simulink model "Distribution_v2"  (Simulink 7.9)
settings: Solver=VariableStepDiscrete  StartTime=0.0  StopTime=1000  RelTol=1e-3
libraries: simeventslib x35
(part 4 of 6)

== system Distribution_v2/Transportation_Channel_42 ==
  note: RESOURCE1 OUTBOUND
      | RESOURCE2 INBOUND
  note: RESOURCE1 INBOUND
      | RESOURCE2 OUTBOUND
  Enabled Gate : EnabledGate
  Enabled Gate1 : EnabledGate
  FIFO Queue : FIFOQueue  Capacity=inf  StatNumberInBlock=on
      settings: OutputPortMap=o1
  FIFO Queue1 : FIFOQueue  Capacity=inf  StatNumberInBlock=on
      settings: OutputPortMap=o1
  Inbound_Process_1 : InfiniteServer  ServiceTimeFrom=Signal port t  ServiceTime=(76.7)/30  StatNumberDeparted=on  StatNumberInBlock=on
      settings: OutputPortMap=o0,o1
  Inbound_Process_2 : InfiniteServer  ServiceTimeFrom=Signal port t  ServiceTime=(76.7)/30  StatNumberDeparted=on  StatNumberInBlock=on
      settings: OutputPortMap=o0,o1
  Inbound_Release_1 : SingleServer  ServiceTime=0  StatNumberInBlock=on
      settings: OutputPortMap=o1
  Inbound_Release_2 : SingleServer  ServiceTime=0  StatNumberInBlock=on
      settings: OutputPortMap=o1
  Infinite Server : InfiniteServer  ServiceTimeFrom=Signal port t  ServiceTime=(76.7)/30
  Infinite Server1 : InfiniteServer  ServiceTimeFrom=Signal port t  ServiceTime=(76.7)/30
  Mux : Mux  Inputs=3
  Outbound_Process_1 : InfiniteServer  ServiceTimeFrom=Signal port t  ServiceTime=(76.7)/30  StatNumberInBlock=on
      settings: OutputPortMap=o1
  Outbound_Process_2 : InfiniteServer  ServiceTimeFrom=Signal port t  ServiceTime=(76.7)/30  StatNumberInBlock=on
      settings: OutputPortMap=o1
  Outbound_Release_1 : SingleServer  ServiceTime=0  StatNumberInBlock=on
      settings: OutputPortMap=o1
  Outbound_Release_2 : SingleServer  ServiceTime=0  StatNumberInBlock=on
      settings: OutputPortMap=o1
  Sum{,1..2,4} (4 alike) : Sum  Inputs=|++
  Sum3 : Sum  Inputs=|++++
  TC_Status : simeventslib/SimEvents Sinks/Discrete Event Signal to Workspace  VariableName=Transportation_Channel_42_Status  SaveFormat=Structure With Time  isMonitorOnly=off  isRecordIC=off
  Timed to Event Signal : TimedToEventSignal
  TravelTime : Constant  Value=139.443/30
  IN_Shipment_1 : PMIOPort  Port=1  Side=Left
  OUT_Shipment_1 : PMIOPort  Port=2  Side=Right
  IN_Resource_1 : PMIOPort  Port=3  Side=Left
  OUT_Resource_1 : PMIOPort  Port=4  Side=Right
  IN_Shipment_2 : PMIOPort  Port=5  Side=Left
  OUT_Shipment_2 : PMIOPort  Port=6  Side=Right
  IN_Resource_2 : PMIOPort  Port=7  Side=Left
  OUT_Resource_2 : PMIOPort  Port=8  Side=Right
  tag scope: Transportation_Channel_42_Status=global
  wires:
  Sum4/1 -> Mux/3
  Inbound_Process_2/1 -> Sum4/2
  Inbound_Process_1/1 -> Sum4/1
  Inbound_Process_2/2 -> Sum3/4
  Outbound_Process_2/1 -> Sum3/3
  Inbound_Process_1/2 -> Sum3/2
  Outbound_Process_1/1 -> Sum3/1
  Sum3/1 -> Mux/2
  Sum/1 -> Mux/1
  Mux/1 -> TC_Status/1, [Transportation_Channel_42_Status]
  Inbound_Release_2/1 -> Sum2/2
  Outbound_Release_1/1 -> Sum2/1
  Sum2/1 -> Enabled Gate/1
  Inbound_Release_1/1 -> Sum1/1
  Outbound_Release_2/1 -> Sum1/2
  Sum1/1 -> Enabled Gate1/1
  Timed to Event Signal/1 -> Infinite Server/1, Inbound_Process_2/1, Inbound_Process_1/1, Infinite Server1/1, Outbound_Process_2/1, Outbound_Process_1/1
  TravelTime/1 -> Timed to Event Signal/1
  FIFO Queue/1 -> Sum/1
  FIFO Queue1/1 -> Sum/2
  connections:
  Inbound_Process_1/RConn1 -- OUT_Resource_1/RConn1
  Outbound_Process_1/RConn1 -- Inbound_Release_1/LConn1
  Inbound_Release_1/RConn1 -- Inbound_Process_1/LConn1
  Outbound_Release_1/RConn1 -- Outbound_Process_1/LConn1
  Inbound_Process_2/RConn1 -- OUT_Resource_2/RConn1
  Inbound_Release_2/RConn1 -- Inbound_Process_2/LConn1
  Outbound_Process_2/RConn1 -- Inbound_Release_2/LConn1
  Outbound_Release_2/RConn1 -- Outbound_Process_2/LConn1
  IN_Resource_2/RConn1 -- Outbound_Release_2/LConn1
  Infinite Server1/RConn1 -- OUT_Shipment_1/RConn1
  Enabled Gate/RConn1 -- Infinite Server1/LConn1
  Infinite Server/LConn1 -- Enabled Gate1/RConn1
  OUT_Shipment_2/RConn1 -- Infinite Server/RConn1
  IN_Resource_1/RConn1 -- Outbound_Release_1/LConn1
  IN_Shipment_2/RConn1 -- FIFO Queue1/LConn1
  IN_Shipment_1/RConn1 -- FIFO Queue/LConn1
  Enabled Gate1/LConn1 -- FIFO Queue1/RConn1
  FIFO Queue/RConn1 -- Enabled Gate/LConn1

== system Distribution_v2/Transportation_Channel_43 ==
  note: RESOURCE1 OUTBOUND
      | RESOURCE2 INBOUND
  note: RESOURCE1 INBOUND
      | RESOURCE2 OUTBOUND
  Enabled Gate : EnabledGate
  Enabled Gate1 : EnabledGate
  FIFO Queue : FIFOQueue  Capacity=inf  StatNumberInBlock=on
      settings: OutputPortMap=o1
  FIFO Queue1 : FIFOQueue  Capacity=inf  StatNumberInBlock=on
      settings: OutputPortMap=o1
  Inbound_Process_1 : InfiniteServer  ServiceTimeFrom=Signal port t  ServiceTime=(76.7)/30  StatNumberDeparted=on  StatNumberInBlock=on
      settings: OutputPortMap=o0,o1
  Inbound_Process_2 : InfiniteServer  ServiceTimeFrom=Signal port t  ServiceTime=(76.7)/30  StatNumberDeparted=on  StatNumberInBlock=on
      settings: OutputPortMap=o0,o1
  Inbound_Release_1 : SingleServer  ServiceTime=0  StatNumberInBlock=on
      settings: OutputPortMap=o1
  Inbound_Release_2 : SingleServer  ServiceTime=0  StatNumberInBlock=on
      settings: OutputPortMap=o1
  Infinite Server : InfiniteServer  ServiceTimeFrom=Signal port t  ServiceTime=(76.7)/30
  Infinite Server1 : InfiniteServer  ServiceTimeFrom=Signal port t  ServiceTime=(76.7)/30
  Mux : Mux  Inputs=3
  Outbound_Process_1 : InfiniteServer  ServiceTimeFrom=Signal port t  ServiceTime=(76.7)/30  StatNumberInBlock=on
      settings: OutputPortMap=o1
  Outbound_Process_2 : InfiniteServer  ServiceTimeFrom=Signal port t  ServiceTime=(76.7)/30  StatNumberInBlock=on
      settings: OutputPortMap=o1
  Outbound_Release_1 : SingleServer  ServiceTime=0  StatNumberInBlock=on
      settings: OutputPortMap=o1
  Outbound_Release_2 : SingleServer  ServiceTime=0  StatNumberInBlock=on
      settings: OutputPortMap=o1
  Sum{,1..2,4} (4 alike) : Sum  Inputs=|++
  Sum3 : Sum  Inputs=|++++
  TC_Status : simeventslib/SimEvents Sinks/Discrete Event Signal to Workspace  VariableName=Transportation_Channel_43_Status  SaveFormat=Structure With Time  isMonitorOnly=off  isRecordIC=off
  Timed to Event Signal : TimedToEventSignal
  TravelTime : Constant  Value=80.2779/30
  IN_Shipment_1 : PMIOPort  Port=1  Side=Left
  OUT_Shipment_1 : PMIOPort  Port=2  Side=Right
  IN_Resource_1 : PMIOPort  Port=3  Side=Left
  OUT_Resource_1 : PMIOPort  Port=4  Side=Right
  IN_Shipment_2 : PMIOPort  Port=5  Side=Left
  OUT_Shipment_2 : PMIOPort  Port=6  Side=Right
  IN_Resource_2 : PMIOPort  Port=7  Side=Left
  OUT_Resource_2 : PMIOPort  Port=8  Side=Right
  tag scope: Transportation_Channel_43_Status=global
  wires:
  Sum4/1 -> Mux/3
  Inbound_Process_2/1 -> Sum4/2
  Inbound_Process_1/1 -> Sum4/1
  Inbound_Process_2/2 -> Sum3/4
  Outbound_Process_2/1 -> Sum3/3
  Inbound_Process_1/2 -> Sum3/2
  Outbound_Process_1/1 -> Sum3/1
  Sum3/1 -> Mux/2
  Sum/1 -> Mux/1
  Mux/1 -> TC_Status/1, [Transportation_Channel_43_Status]
  Inbound_Release_2/1 -> Sum2/2
  Outbound_Release_1/1 -> Sum2/1
  Sum2/1 -> Enabled Gate/1
  Inbound_Release_1/1 -> Sum1/1
  Outbound_Release_2/1 -> Sum1/2
  Sum1/1 -> Enabled Gate1/1
  Timed to Event Signal/1 -> Infinite Server/1, Inbound_Process_2/1, Inbound_Process_1/1, Infinite Server1/1, Outbound_Process_2/1, Outbound_Process_1/1
  TravelTime/1 -> Timed to Event Signal/1
  FIFO Queue/1 -> Sum/1
  FIFO Queue1/1 -> Sum/2
  connections:
  Inbound_Process_1/RConn1 -- OUT_Resource_1/RConn1
  Outbound_Process_1/RConn1 -- Inbound_Release_1/LConn1
  Inbound_Release_1/RConn1 -- Inbound_Process_1/LConn1
  Outbound_Release_1/RConn1 -- Outbound_Process_1/LConn1
  Inbound_Process_2/RConn1 -- OUT_Resource_2/RConn1
  Inbound_Release_2/RConn1 -- Inbound_Process_2/LConn1
  Outbound_Process_2/RConn1 -- Inbound_Release_2/LConn1
  Outbound_Release_2/RConn1 -- Outbound_Process_2/LConn1
  IN_Resource_2/RConn1 -- Outbound_Release_2/LConn1
  Infinite Server1/RConn1 -- OUT_Shipment_1/RConn1
  Enabled Gate/RConn1 -- Infinite Server1/LConn1
  Infinite Server/LConn1 -- Enabled Gate1/RConn1
  OUT_Shipment_2/RConn1 -- Infinite Server/RConn1
  IN_Resource_1/RConn1 -- Outbound_Release_1/LConn1
  IN_Shipment_2/RConn1 -- FIFO Queue1/LConn1
  IN_Shipment_1/RConn1 -- FIFO Queue/LConn1
  Enabled Gate1/LConn1 -- FIFO Queue1/RConn1
  FIFO Queue/RConn1 -- Enabled Gate/LConn1

== system Distribution_v2/Transportation_Channel_44 ==
  note: RESOURCE1 OUTBOUND
      | RESOURCE2 INBOUND
  note: RESOURCE1 INBOUND
      | RESOURCE2 OUTBOUND
  Enabled Gate : EnabledGate
  Enabled Gate1 : EnabledGate
  FIFO Queue : FIFOQueue  Capacity=inf  StatNumberInBlock=on
      settings: OutputPortMap=o1
  FIFO Queue1 : FIFOQueue  Capacity=inf  StatNumberInBlock=on
      settings: OutputPortMap=o1
  Inbound_Process_1 : InfiniteServer  ServiceTimeFrom=Signal port t  ServiceTime=(76.7)/30  StatNumberDeparted=on  StatNumberInBlock=on
      settings: OutputPortMap=o0,o1
  Inbound_Process_2 : InfiniteServer  ServiceTimeFrom=Signal port t  ServiceTime=(76.7)/30  StatNumberDeparted=on  StatNumberInBlock=on
      settings: OutputPortMap=o0,o1
  Inbound_Release_1 : SingleServer  ServiceTime=0  StatNumberInBlock=on
      settings: OutputPortMap=o1
  Inbound_Release_2 : SingleServer  ServiceTime=0  StatNumberInBlock=on
      settings: OutputPortMap=o1
  Infinite Server : InfiniteServer  ServiceTimeFrom=Signal port t  ServiceTime=(76.7)/30
  Infinite Server1 : InfiniteServer  ServiceTimeFrom=Signal port t  ServiceTime=(76.7)/30
  Mux : Mux  Inputs=3
  Outbound_Process_1 : InfiniteServer  ServiceTimeFrom=Signal port t  ServiceTime=(76.7)/30  StatNumberInBlock=on
      settings: OutputPortMap=o1
  Outbound_Process_2 : InfiniteServer  ServiceTimeFrom=Signal port t  ServiceTime=(76.7)/30  StatNumberInBlock=on
      settings: OutputPortMap=o1
  Outbound_Release_1 : SingleServer  ServiceTime=0  StatNumberInBlock=on
      settings: OutputPortMap=o1
  Outbound_Release_2 : SingleServer  ServiceTime=0  StatNumberInBlock=on
      settings: OutputPortMap=o1
  Sum{,1..2,4} (4 alike) : Sum  Inputs=|++
  Sum3 : Sum  Inputs=|++++
  TC_Status : simeventslib/SimEvents Sinks/Discrete Event Signal to Workspace  VariableName=Transportation_Channel_44_Status  SaveFormat=Structure With Time  isMonitorOnly=off  isRecordIC=off
  Timed to Event Signal : TimedToEventSignal
  TravelTime : Constant  Value=93.9426/30
  IN_Shipment_1 : PMIOPort  Port=1  Side=Left
  OUT_Shipment_1 : PMIOPort  Port=2  Side=Right
  IN_Resource_1 : PMIOPort  Port=3  Side=Left
  OUT_Resource_1 : PMIOPort  Port=4  Side=Right
  IN_Shipment_2 : PMIOPort  Port=5  Side=Left
  OUT_Shipment_2 : PMIOPort  Port=6  Side=Right
  IN_Resource_2 : PMIOPort  Port=7  Side=Left
  OUT_Resource_2 : PMIOPort  Port=8  Side=Right
  tag scope: Transportation_Channel_44_Status=global
  wires:
  Sum4/1 -> Mux/3
  Inbound_Process_2/1 -> Sum4/2
  Inbound_Process_1/1 -> Sum4/1
  Inbound_Process_2/2 -> Sum3/4
  Outbound_Process_2/1 -> Sum3/3
  Inbound_Process_1/2 -> Sum3/2
  Outbound_Process_1/1 -> Sum3/1
  Sum3/1 -> Mux/2
  Sum/1 -> Mux/1
  Mux/1 -> TC_Status/1, [Transportation_Channel_44_Status]
  Inbound_Release_2/1 -> Sum2/2
  Outbound_Release_1/1 -> Sum2/1
  Sum2/1 -> Enabled Gate/1
  Inbound_Release_1/1 -> Sum1/1
  Outbound_Release_2/1 -> Sum1/2
  Sum1/1 -> Enabled Gate1/1
  Timed to Event Signal/1 -> Infinite Server/1, Inbound_Process_2/1, Inbound_Process_1/1, Infinite Server1/1, Outbound_Process_2/1, Outbound_Process_1/1
  TravelTime/1 -> Timed to Event Signal/1
  FIFO Queue/1 -> Sum/1
  FIFO Queue1/1 -> Sum/2
  connections:
  Inbound_Process_1/RConn1 -- OUT_Resource_1/RConn1
  Outbound_Process_1/RConn1 -- Inbound_Release_1/LConn1
  Inbound_Release_1/RConn1 -- Inbound_Process_1/LConn1
  Outbound_Release_1/RConn1 -- Outbound_Process_1/LConn1
  Inbound_Process_2/RConn1 -- OUT_Resource_2/RConn1
  Inbound_Release_2/RConn1 -- Inbound_Process_2/LConn1
  Outbound_Process_2/RConn1 -- Inbound_Release_2/LConn1
  Outbound_Release_2/RConn1 -- Outbound_Process_2/LConn1
  IN_Resource_2/RConn1 -- Outbound_Release_2/LConn1
  Infinite Server1/RConn1 -- OUT_Shipment_1/RConn1
  Enabled Gate/RConn1 -- Infinite Server1/LConn1
  Infinite Server/LConn1 -- Enabled Gate1/RConn1
  OUT_Shipment_2/RConn1 -- Infinite Server/RConn1
  IN_Resource_1/RConn1 -- Outbound_Release_1/LConn1
  IN_Shipment_2/RConn1 -- FIFO Queue1/LConn1
  IN_Shipment_1/RConn1 -- FIFO Queue/LConn1
  Enabled Gate1/LConn1 -- FIFO Queue1/RConn1
  FIFO Queue/RConn1 -- Enabled Gate/LConn1

== system Distribution_v2/Transportation_Channel_45 ==
  note: RESOURCE1 OUTBOUND
      | RESOURCE2 INBOUND
  note: RESOURCE1 INBOUND
      | RESOURCE2 OUTBOUND
  Enabled Gate : EnabledGate
  Enabled Gate1 : EnabledGate
  FIFO Queue : FIFOQueue  Capacity=inf  StatNumberInBlock=on
      settings: OutputPortMap=o1
  FIFO Queue1 : FIFOQueue  Capacity=inf  StatNumberInBlock=on
      settings: OutputPortMap=o1
  Inbound_Process_1 : InfiniteServer  ServiceTimeFrom=Signal port t  ServiceTime=(76.7)/30  StatNumberDeparted=on  StatNumberInBlock=on
      settings: OutputPortMap=o0,o1
  Inbound_Process_2 : InfiniteServer  ServiceTimeFrom=Signal port t  ServiceTime=(76.7)/30  StatNumberDeparted=on  StatNumberInBlock=on
      settings: OutputPortMap=o0,o1
  Inbound_Release_1 : SingleServer  ServiceTime=0  StatNumberInBlock=on
      settings: OutputPortMap=o1
  Inbound_Release_2 : SingleServer  ServiceTime=0  StatNumberInBlock=on
      settings: OutputPortMap=o1
  Infinite Server : InfiniteServer  ServiceTimeFrom=Signal port t  ServiceTime=(76.7)/30
  Infinite Server1 : InfiniteServer  ServiceTimeFrom=Signal port t  ServiceTime=(76.7)/30
  Mux : Mux  Inputs=3
  Outbound_Process_1 : InfiniteServer  ServiceTimeFrom=Signal port t  ServiceTime=(76.7)/30  StatNumberInBlock=on
      settings: OutputPortMap=o1
  Outbound_Process_2 : InfiniteServer  ServiceTimeFrom=Signal port t  ServiceTime=(76.7)/30  StatNumberInBlock=on
      settings: OutputPortMap=o1
  Outbound_Release_1 : SingleServer  ServiceTime=0  StatNumberInBlock=on
      settings: OutputPortMap=o1
  Outbound_Release_2 : SingleServer  ServiceTime=0  StatNumberInBlock=on
      settings: OutputPortMap=o1
  Sum{,1..2,4} (4 alike) : Sum  Inputs=|++
  Sum3 : Sum  Inputs=|++++
  TC_Status : simeventslib/SimEvents Sinks/Discrete Event Signal to Workspace  VariableName=Transportation_Channel_45_Status  SaveFormat=Structure With Time  isMonitorOnly=off  isRecordIC=off
  Timed to Event Signal : TimedToEventSignal
  TravelTime : Constant  Value=80.6308/30
  IN_Shipment_1 : PMIOPort  Port=1  Side=Left
  OUT_Shipment_1 : PMIOPort  Port=2  Side=Right
  IN_Resource_1 : PMIOPort  Port=3  Side=Left
  OUT_Resource_1 : PMIOPort  Port=4  Side=Right
  IN_Shipment_2 : PMIOPort  Port=5  Side=Left
  OUT_Shipment_2 : PMIOPort  Port=6  Side=Right
  IN_Resource_2 : PMIOPort  Port=7  Side=Left
  OUT_Resource_2 : PMIOPort  Port=8  Side=Right
  tag scope: Transportation_Channel_45_Status=global
  wires:
  Sum4/1 -> Mux/3
  Inbound_Process_2/1 -> Sum4/2
  Inbound_Process_1/1 -> Sum4/1
  Inbound_Process_2/2 -> Sum3/4
  Outbound_Process_2/1 -> Sum3/3
  Inbound_Process_1/2 -> Sum3/2
  Outbound_Process_1/1 -> Sum3/1
  Sum3/1 -> Mux/2
  Sum/1 -> Mux/1
  Mux/1 -> TC_Status/1, [Transportation_Channel_45_Status]
  Inbound_Release_2/1 -> Sum2/2
  Outbound_Release_1/1 -> Sum2/1
  Sum2/1 -> Enabled Gate/1
  Inbound_Release_1/1 -> Sum1/1
  Outbound_Release_2/1 -> Sum1/2
  Sum1/1 -> Enabled Gate1/1
  Timed to Event Signal/1 -> Infinite Server/1, Inbound_Process_2/1, Inbound_Process_1/1, Infinite Server1/1, Outbound_Process_2/1, Outbound_Process_1/1
  TravelTime/1 -> Timed to Event Signal/1
  FIFO Queue/1 -> Sum/1
  FIFO Queue1/1 -> Sum/2
  connections:
  Inbound_Process_1/RConn1 -- OUT_Resource_1/RConn1
  Outbound_Process_1/RConn1 -- Inbound_Release_1/LConn1
  Inbound_Release_1/RConn1 -- Inbound_Process_1/LConn1
  Outbound_Release_1/RConn1 -- Outbound_Process_1/LConn1
  Inbound_Process_2/RConn1 -- OUT_Resource_2/RConn1
  Inbound_Release_2/RConn1 -- Inbound_Process_2/LConn1
  Outbound_Process_2/RConn1 -- Inbound_Release_2/LConn1
  Outbound_Release_2/RConn1 -- Outbound_Process_2/LConn1
  IN_Resource_2/RConn1 -- Outbound_Release_2/LConn1
  Infinite Server1/RConn1 -- OUT_Shipment_1/RConn1
  Enabled Gate/RConn1 -- Infinite Server1/LConn1
  Infinite Server/LConn1 -- Enabled Gate1/RConn1
  OUT_Shipment_2/RConn1 -- Infinite Server/RConn1
  IN_Resource_1/RConn1 -- Outbound_Release_1/LConn1
  IN_Shipment_2/RConn1 -- FIFO Queue1/LConn1
  IN_Shipment_1/RConn1 -- FIFO Queue/LConn1
  Enabled Gate1/LConn1 -- FIFO Queue1/RConn1
  FIFO Queue/RConn1 -- Enabled Gate/LConn1

== system Distribution_v2/Customer_1/Commodity_1 ==
  Clock : Clock
  Source : TimeBasedEntityGenerator  Distribution=Exponential  InitialSeed=18340  Mean=Mean  GenerateEntityAtSimulationStart=off
  Timed to Event Signal : TimedToEventSignal
  setAttribute : SetAttribute  AttributeName=Route|Origin|Destination|Start  AttributeFrom=Dialog|Dialog|Dialog|Signal port  AttributeValue="[1  22  18   2]|1|2|1"  AttributeTreatAsVector=0|1|1|1  EvaluatedAttributeValue="{[1  22  18   2];1;2;[]}"
      settings: InputPortMap=u3
  OUT_Commodity : PMIOPort  Port=1  Side=Right
  wires:
  Timed to Event Signal/1 -> setAttribute/1
  Clock/1 -> Timed to Event Signal/1
  connections:
  OUT_Commodity/RConn1 -- setAttribute/RConn1
  Source/RConn1 -- setAttribute/LConn1

== system Distribution_v2/Customer_1/Commodity_2 ==
  Clock : Clock
  Source : TimeBasedEntityGenerator  Distribution=Exponential  InitialSeed=18340  Mean=Mean  GenerateEntityAtSimulationStart=off
  Timed to Event Signal : TimedToEventSignal
  setAttribute : SetAttribute  AttributeName=Route|Origin|Destination|Start  AttributeFrom=Dialog|Dialog|Dialog|Signal port  AttributeValue="[1  22  18   4]|1|4|1"  AttributeTreatAsVector=0|1|1|1  EvaluatedAttributeValue="{[1  22  18   4];1;4;[]}"
      settings: InputPortMap=u3
  OUT_Commodity : PMIOPort  Port=1  Side=Right
  wires:
  Timed to Event Signal/1 -> setAttribute/1
  Clock/1 -> Timed to Event Signal/1
  connections:
  OUT_Commodity/RConn1 -- setAttribute/RConn1
  Source/RConn1 -- setAttribute/LConn1

== system Distribution_v2/Customer_1/Commodity_3 ==
  Clock : Clock
  Source : TimeBasedEntityGenerator  Distribution=Exponential  InitialSeed=18340  Mean=Mean  GenerateEntityAtSimulationStart=off
  Timed to Event Signal : TimedToEventSignal
  setAttribute : SetAttribute  AttributeName=Route|Origin|Destination|Start  AttributeFrom=Dialog|Dialog|Dialog|Signal port  AttributeValue="[1  22   5   0]|1|5|1"  AttributeTreatAsVector=0|1|1|1  EvaluatedAttributeValue="{[1  22   5   0];1;5;[]}"
      settings: InputPortMap=u3
  OUT_Commodity : PMIOPort  Port=1  Side=Right
  wires:
  Timed to Event Signal/1 -> setAttribute/1
  Clock/1 -> Timed to Event Signal/1
  connections:
  OUT_Commodity/RConn1 -- setAttribute/RConn1
  Source/RConn1 -- setAttribute/LConn1

== system Distribution_v2/Customer_1/Commodity_4 ==
  Clock : Clock
  Source : TimeBasedEntityGenerator  Distribution=Exponential  InitialSeed=18340  Mean=Mean  GenerateEntityAtSimulationStart=off
  Timed to Event Signal : TimedToEventSignal
  setAttribute : SetAttribute  AttributeName=Route|Origin|Destination|Start  AttributeFrom=Dialog|Dialog|Dialog|Signal port  AttributeValue="[1  22  18   6]|1|6|1"  AttributeTreatAsVector=0|1|1|1  EvaluatedAttributeValue="{[1  22  18   6];1;6;[]}"
      settings: InputPortMap=u3
  OUT_Commodity : PMIOPort  Port=1  Side=Right
  wires:
  Timed to Event Signal/1 -> setAttribute/1
  Clock/1 -> Timed to Event Signal/1
  connections:
  OUT_Commodity/RConn1 -- setAttribute/RConn1
  Source/RConn1 -- setAttribute/LConn1

== system Distribution_v2/Customer_1/Commodity_5 ==
  Clock : Clock
  Source : TimeBasedEntityGenerator  Distribution=Exponential  InitialSeed=18340  Mean=Mean  GenerateEntityAtSimulationStart=off
  Timed to Event Signal : TimedToEventSignal
  setAttribute : SetAttribute  AttributeName=Route|Origin|Destination|Start  AttributeFrom=Dialog|Dialog|Dialog|Signal port  AttributeValue="[1  22  20   7]|1|7|1"  AttributeTreatAsVector=0|1|1|1  EvaluatedAttributeValue="{[1  22  20   7];1;7;[]}"
      settings: InputPortMap=u3
  OUT_Commodity : PMIOPort  Port=1  Side=Right
  wires:
  Timed to Event Signal/1 -> setAttribute/1
  Clock/1 -> Timed to Event Signal/1
  connections:
  OUT_Commodity/RConn1 -- setAttribute/RConn1
  Source/RConn1 -- setAttribute/LConn1

== system Distribution_v2/Customer_1/Commodity_6 ==
  Clock : Clock
  Source : TimeBasedEntityGenerator  Distribution=Exponential  InitialSeed=18340  Mean=Mean  GenerateEntityAtSimulationStart=off
  Timed to Event Signal : TimedToEventSignal
  setAttribute : SetAttribute  AttributeName=Route|Origin|Destination|Start  AttributeFrom=Dialog|Dialog|Dialog|Signal port  AttributeValue="[1  22  20   8]|1|8|1"  AttributeTreatAsVector=0|1|1|1  EvaluatedAttributeValue="{[1  22  20   8];1;8;[]}"
      settings: InputPortMap=u3
  OUT_Commodity : PMIOPort  Port=1  Side=Right
  wires:
  Timed to Event Signal/1 -> setAttribute/1
  Clock/1 -> Timed to Event Signal/1
  connections:
  OUT_Commodity/RConn1 -- setAttribute/RConn1
  Source/RConn1 -- setAttribute/LConn1

== system Distribution_v2/Customer_1/Commodity_7 ==
  Clock : Clock
  Source : TimeBasedEntityGenerator  Distribution=Exponential  InitialSeed=18340  Mean=Mean  GenerateEntityAtSimulationStart=off
  Timed to Event Signal : TimedToEventSignal
  setAttribute : SetAttribute  AttributeName=Route|Origin|Destination|Start  AttributeFrom=Dialog|Dialog|Dialog|Signal port  AttributeValue="[1  22  13   0]|1|13|1"  AttributeTreatAsVector=0|1|1|1  EvaluatedAttributeValue="{[1  22  13   0];1;13;[]}"
      settings: InputPortMap=u3
  OUT_Commodity : PMIOPort  Port=1  Side=Right
  wires:
  Timed to Event Signal/1 -> setAttribute/1
  Clock/1 -> Timed to Event Signal/1
  connections:
  OUT_Commodity/RConn1 -- setAttribute/RConn1
  Source/RConn1 -- setAttribute/LConn1

== system Distribution_v2/Customer_1/Commodity_8 ==
  Clock : Clock
  Source : TimeBasedEntityGenerator  Distribution=Exponential  InitialSeed=18340  Mean=Mean  GenerateEntityAtSimulationStart=off
  Timed to Event Signal : TimedToEventSignal
  setAttribute : SetAttribute  AttributeName=Route|Origin|Destination|Start  AttributeFrom=Dialog|Dialog|Dialog|Signal port  AttributeValue="[1  22  20  14]|1|14|1"  AttributeTreatAsVector=0|1|1|1  EvaluatedAttributeValue="{[1  22  20  14];1;14;[]}"
      settings: InputPortMap=u3
  OUT_Commodity : PMIOPort  Port=1  Side=Right
  wires:
  Timed to Event Signal/1 -> setAttribute/1
  Clock/1 -> Timed to Event Signal/1
  connections:
  OUT_Commodity/RConn1 -- setAttribute/RConn1
  Source/RConn1 -- setAttribute/LConn1

== system Distribution_v2/Customer_1/Commodity_9 ==
  Clock : Clock
  Source : TimeBasedEntityGenerator  Distribution=Exponential  InitialSeed=18340  Mean=Mean  GenerateEntityAtSimulationStart=off
  Timed to Event Signal : TimedToEventSignal
  setAttribute : SetAttribute  AttributeName=Route|Origin|Destination|Start  AttributeFrom=Dialog|Dialog|Dialog|Signal port  AttributeValue="[1  22  20  15]|1|15|1"  AttributeTreatAsVector=0|1|1|1  EvaluatedAttributeValue="{[1  22  20  15];1;15;[]}"
      settings: InputPortMap=u3
  OUT_Commodity : PMIOPort  Port=1  Side=Right
  wires:
  Timed to Event Signal/1 -> setAttribute/1
  Clock/1 -> Timed to Event Signal/1
  connections:
  OUT_Commodity/RConn1 -- setAttribute/RConn1
  Source/RConn1 -- setAttribute/LConn1

== system Distribution_v2/Customer_10/Commodity_75 ==
  Clock : Clock
  Source : TimeBasedEntityGenerator  Distribution=Exponential  InitialSeed=18340  Mean=Mean  GenerateEntityAtSimulationStart=off
  Timed to Event Signal : TimedToEventSignal
  setAttribute : SetAttribute  AttributeName=Route|Origin|Destination|Start  AttributeFrom=Dialog|Dialog|Dialog|Signal port  AttributeValue="[10  22  18   4]|10|4|1"  AttributeTreatAsVector=0|1|1|1  EvaluatedAttributeValue="{[10  22  18   4];10;4;[]}"
      settings: InputPortMap=u3
  OUT_Commodity : PMIOPort  Port=1  Side=Right
  wires:
  Timed to Event Signal/1 -> setAttribute/1
  Clock/1 -> Timed to Event Signal/1
  connections:
  OUT_Commodity/RConn1 -- setAttribute/RConn1
  Source/RConn1 -- setAttribute/LConn1

== system Distribution_v2/Customer_10/Commodity_76 ==
  Clock : Clock
  Source : TimeBasedEntityGenerator  Distribution=Exponential  InitialSeed=18340  Mean=Mean  GenerateEntityAtSimulationStart=off
  Timed to Event Signal : TimedToEventSignal
  setAttribute : SetAttribute  AttributeName=Route|Origin|Destination|Start  AttributeFrom=Dialog|Dialog|Dialog|Signal port  AttributeValue="[10  22  20   7]|10|7|1"  AttributeTreatAsVector=0|1|1|1  EvaluatedAttributeValue="{[10  22  20   7];10;7;[]}"
      settings: InputPortMap=u3
  OUT_Commodity : PMIOPort  Port=1  Side=Right
  wires:
  Timed to Event Signal/1 -> setAttribute/1
  Clock/1 -> Timed to Event Signal/1
  connections:
  OUT_Commodity/RConn1 -- setAttribute/RConn1
  Source/RConn1 -- setAttribute/LConn1

== system Distribution_v2/Customer_10/Commodity_77 ==
  Clock : Clock
  Source : TimeBasedEntityGenerator  Distribution=Exponential  InitialSeed=18340  Mean=Mean  GenerateEntityAtSimulationStart=off
  Timed to Event Signal : TimedToEventSignal
  setAttribute : SetAttribute  AttributeName=Route|Origin|Destination|Start  AttributeFrom=Dialog|Dialog|Dialog|Signal port  AttributeValue="[10  22  18   9]|10|9|1"  AttributeTreatAsVector=0|1|1|1  EvaluatedAttributeValue="{[10  22  18   9];10;9;[]}"
      settings: InputPortMap=u3
  OUT_Commodity : PMIOPort  Port=1  Side=Right
  wires:
  Timed to Event Signal/1 -> setAttribute/1
  Clock/1 -> Timed to Event Signal/1
  connections:
  OUT_Commodity/RConn1 -- setAttribute/RConn1
  Source/RConn1 -- setAttribute/LConn1

== system Distribution_v2/Customer_10/Commodity_78 ==
  Clock : Clock
  Source : TimeBasedEntityGenerator  Distribution=Exponential  InitialSeed=18340  Mean=Mean  GenerateEntityAtSimulationStart=off
  Timed to Event Signal : TimedToEventSignal
  setAttribute : SetAttribute  AttributeName=Route|Origin|Destination|Start  AttributeFrom=Dialog|Dialog|Dialog|Signal port  AttributeValue="[10  22  13   0]|10|13|1"  AttributeTreatAsVector=0|1|1|1  EvaluatedAttributeValue="{[10  22  13   0];10;13;[]}"
      settings: InputPortMap=u3
  OUT_Commodity : PMIOPort  Port=1  Side=Right
  wires:
  Timed to Event Signal/1 -> setAttribute/1
  Clock/1 -> Timed to Event Signal/1
  connections:
  OUT_Commodity/RConn1 -- setAttribute/RConn1
  Source/RConn1 -- setAttribute/LConn1

== system Distribution_v2/Customer_10/Commodity_79 ==
  Clock : Clock
  Source : TimeBasedEntityGenerator  Distribution=Exponential  InitialSeed=18340  Mean=Mean  GenerateEntityAtSimulationStart=off
  Timed to Event Signal : TimedToEventSignal
  setAttribute : SetAttribute  AttributeName=Route|Origin|Destination|Start  AttributeFrom=Dialog|Dialog|Dialog|Signal port  AttributeValue="[10  22  20  14]|10|14|1"  AttributeTreatAsVector=0|1|1|1  EvaluatedAttributeValue="{[10  22  20  14];10;14;[]}"
      settings: InputPortMap=u3
  OUT_Commodity : PMIOPort  Port=1  Side=Right
  wires:
  Timed to Event Signal/1 -> setAttribute/1
  Clock/1 -> Timed to Event Signal/1
  connections:
  OUT_Commodity/RConn1 -- setAttribute/RConn1
  Source/RConn1 -- setAttribute/LConn1

== system Distribution_v2/Customer_10/Commodity_80 ==
  Clock : Clock
  Source : TimeBasedEntityGenerator  Distribution=Exponential  InitialSeed=18340  Mean=Mean  GenerateEntityAtSimulationStart=off
  Timed to Event Signal : TimedToEventSignal
  setAttribute : SetAttribute  AttributeName=Route|Origin|Destination|Start  AttributeFrom=Dialog|Dialog|Dialog|Signal port  AttributeValue="[10  22  20  15]|10|15|1"  AttributeTreatAsVector=0|1|1|1  EvaluatedAttributeValue="{[10  22  20  15];10;15;[]}"
      settings: InputPortMap=u3
  OUT_Commodity : PMIOPort  Port=1  Side=Right
  wires:
  Timed to Event Signal/1 -> setAttribute/1
  Clock/1 -> Timed to Event Signal/1
  connections:
  OUT_Commodity/RConn1 -- setAttribute/RConn1
  Source/RConn1 -- setAttribute/LConn1

== system Distribution_v2/Customer_11/Commodity_81 ==
  Clock : Clock
  Source : TimeBasedEntityGenerator  Distribution=Exponential  InitialSeed=18340  Mean=Mean  GenerateEntityAtSimulationStart=off
  Timed to Event Signal : TimedToEventSignal
  setAttribute : SetAttribute  AttributeName=Route|Origin|Destination|Start  AttributeFrom=Dialog|Dialog|Dialog|Signal port  AttributeValue="[11  20  22   1]|11|1|1"  AttributeTreatAsVector=0|1|1|1  EvaluatedAttributeValue="{[11  20  22   1];11;1;[]}"
      settings: InputPortMap=u3
  OUT_Commodity : PMIOPort  Port=1  Side=Right
  wires:
  Timed to Event Signal/1 -> setAttribute/1
  Clock/1 -> Timed to Event Signal/1
  connections:
  OUT_Commodity/RConn1 -- setAttribute/RConn1
  Source/RConn1 -- setAttribute/LConn1

== system Distribution_v2/Customer_11/Commodity_82 ==
  Clock : Clock
  Source : TimeBasedEntityGenerator  Distribution=Exponential  InitialSeed=18340  Mean=Mean  GenerateEntityAtSimulationStart=off
  Timed to Event Signal : TimedToEventSignal
  setAttribute : SetAttribute  AttributeName=Route|Origin|Destination|Start  AttributeFrom=Dialog|Dialog|Dialog|Signal port  AttributeValue="[11  20  18   2]|11|2|1"  AttributeTreatAsVector=0|1|1|1  EvaluatedAttributeValue="{[11  20  18   2];11;2;[]}"
      settings: InputPortMap=u3
  OUT_Commodity : PMIOPort  Port=1  Side=Right
  wires:
  Timed to Event Signal/1 -> setAttribute/1
  Clock/1 -> Timed to Event Signal/1
  connections:
  OUT_Commodity/RConn1 -- setAttribute/RConn1
  Source/RConn1 -- setAttribute/LConn1

== system Distribution_v2/Customer_11/Commodity_83 ==
  Clock : Clock
  Source : TimeBasedEntityGenerator  Distribution=Exponential  InitialSeed=18340  Mean=Mean  GenerateEntityAtSimulationStart=off
  Timed to Event Signal : TimedToEventSignal
  setAttribute : SetAttribute  AttributeName=Route|Origin|Destination|Start  AttributeFrom=Dialog|Dialog|Dialog|Signal port  AttributeValue="[11  20  18   6]|11|6|1"  AttributeTreatAsVector=0|1|1|1  EvaluatedAttributeValue="{[11  20  18   6];11;6;[]}"
      settings: InputPortMap=u3
  OUT_Commodity : PMIOPort  Port=1  Side=Right
  wires:
  Timed to Event Signal/1 -> setAttribute/1
  Clock/1 -> Timed to Event Signal/1
  connections:
  OUT_Commodity/RConn1 -- setAttribute/RConn1
  Source/RConn1 -- setAttribute/LConn1

== system Distribution_v2/Customer_11/Commodity_84 ==
  Clock : Clock
  Source : TimeBasedEntityGenerator  Distribution=Exponential  InitialSeed=18340  Mean=Mean  GenerateEntityAtSimulationStart=off
  Timed to Event Signal : TimedToEventSignal
  setAttribute : SetAttribute  AttributeName=Route|Origin|Destination|Start  AttributeFrom=Dialog|Dialog|Dialog|Signal port  AttributeValue="[11  20   7   0]|11|7|1"  AttributeTreatAsVector=0|1|1|1  EvaluatedAttributeValue="{[11  20   7   0];11;7;[]}"
      settings: InputPortMap=u3
  OUT_Commodity : PMIOPort  Port=1  Side=Right
  wires:
  Timed to Event Signal/1 -> setAttribute/1
  Clock/1 -> Timed to Event Signal/1
  connections:
  OUT_Commodity/RConn1 -- setAttribute/RConn1
  Source/RConn1 -- setAttribute/LConn1

== system Distribution_v2/Customer_11/Commodity_85 ==
  Clock : Clock
  Source : TimeBasedEntityGenerator  Distribution=Exponential  InitialSeed=18340  Mean=Mean  GenerateEntityAtSimulationStart=off
  Timed to Event Signal : TimedToEventSignal
  setAttribute : SetAttribute  AttributeName=Route|Origin|Destination|Start  AttributeFrom=Dialog|Dialog|Dialog|Signal port  AttributeValue="[11  20  22  10]|11|10|1"  AttributeTreatAsVector=0|1|1|1  EvaluatedAttributeValue="{[11  20  22  10];11;10;[]}"
      settings: InputPortMap=u3
  OUT_Commodity : PMIOPort  Port=1  Side=Right
  wires:
  Timed to Event Signal/1 -> setAttribute/1
  Clock/1 -> Timed to Event Signal/1
  connections:
  OUT_Commodity/RConn1 -- setAttribute/RConn1
  Source/RConn1 -- setAttribute/LConn1

== system Distribution_v2/Customer_12/Commodity_86 ==
  Clock : Clock
  Source : TimeBasedEntityGenerator  Distribution=Exponential  InitialSeed=18340  Mean=Mean  GenerateEntityAtSimulationStart=off
  Timed to Event Signal : TimedToEventSignal
  setAttribute : SetAttribute  AttributeName=Route|Origin|Destination|Start  AttributeFrom=Dialog|Dialog|Dialog|Signal port  AttributeValue="[12  22  18   2]|12|2|1"  AttributeTreatAsVector=0|1|1|1  EvaluatedAttributeValue="{[12  22  18   2];12;2;[]}"
      settings: InputPortMap=u3
  OUT_Commodity : PMIOPort  Port=1  Side=Right
  wires:
  Timed to Event Signal/1 -> setAttribute/1
  Clock/1 -> Timed to Event Signal/1
  connections:
  OUT_Commodity/RConn1 -- setAttribute/RConn1
  Source/RConn1 -- setAttribute/LConn1

== system Distribution_v2/Customer_12/Commodity_87 ==
  Clock : Clock
  Source : TimeBasedEntityGenerator  Distribution=Exponential  InitialSeed=18340  Mean=Mean  GenerateEntityAtSimulationStart=off
  Timed to Event Signal : TimedToEventSignal
  setAttribute : SetAttribute  AttributeName=Route|Origin|Destination|Start  AttributeFrom=Dialog|Dialog|Dialog|Signal port  AttributeValue="[12  22  18   4]|12|4|1"  AttributeTreatAsVector=0|1|1|1  EvaluatedAttributeValue="{[12  22  18   4];12;4;[]}"
      settings: InputPortMap=u3
  OUT_Commodity : PMIOPort  Port=1  Side=Right
  wires:
  Timed to Event Signal/1 -> setAttribute/1
  Clock/1 -> Timed to Event Signal/1
  connections:
  OUT_Commodity/RConn1 -- setAttribute/RConn1
  Source/RConn1 -- setAttribute/LConn1

== system Distribution_v2/Customer_12/Commodity_88 ==
  Clock : Clock
  Source : TimeBasedEntityGenerator  Distribution=Exponential  InitialSeed=18340  Mean=Mean  GenerateEntityAtSimulationStart=off
  Timed to Event Signal : TimedToEventSignal
  setAttribute : SetAttribute  AttributeName=Route|Origin|Destination|Start  AttributeFrom=Dialog|Dialog|Dialog|Signal port  AttributeValue="[12  22   5   0]|12|5|1"  AttributeTreatAsVector=0|1|1|1  EvaluatedAttributeValue="{[12  22   5   0];12;5;[]}"
      settings: InputPortMap=u3
  OUT_Commodity : PMIOPort  Port=1  Side=Right
  wires:
  Timed to Event Signal/1 -> setAttribute/1
  Clock/1 -> Timed to Event Signal/1
  connections:
  OUT_Commodity/RConn1 -- setAttribute/RConn1
  Source/RConn1 -- setAttribute/LConn1

== system Distribution_v2/Customer_12/Commodity_89 ==
  Clock : Clock
  Source : TimeBasedEntityGenerator  Distribution=Exponential  InitialSeed=18340  Mean=Mean  GenerateEntityAtSimulationStart=off
  Timed to Event Signal : TimedToEventSignal
  setAttribute : SetAttribute  AttributeName=Route|Origin|Destination|Start  AttributeFrom=Dialog|Dialog|Dialog|Signal port  AttributeValue="[12  22  20   8]|12|8|1"  AttributeTreatAsVector=0|1|1|1  EvaluatedAttributeValue="{[12  22  20   8];12;8;[]}"
      settings: InputPortMap=u3
  OUT_Commodity : PMIOPort  Port=1  Side=Right
  wires:
  Timed to Event Signal/1 -> setAttribute/1
  Clock/1 -> Timed to Event Signal/1
  connections:
  OUT_Commodity/RConn1 -- setAttribute/RConn1
  Source/RConn1 -- setAttribute/LConn1

== system Distribution_v2/Customer_12/Commodity_90 ==
  Clock : Clock
  Source : TimeBasedEntityGenerator  Distribution=Exponential  InitialSeed=18340  Mean=Mean  GenerateEntityAtSimulationStart=off
  Timed to Event Signal : TimedToEventSignal
  setAttribute : SetAttribute  AttributeName=Route|Origin|Destination|Start  AttributeFrom=Dialog|Dialog|Dialog|Signal port  AttributeValue="[12  22  10   0]|12|10|1"  AttributeTreatAsVector=0|1|1|1  EvaluatedAttributeValue="{[12  22  10   0];12;10;[]}"
      settings: InputPortMap=u3
  OUT_Commodity : PMIOPort  Port=1  Side=Right
  wires:
  Timed to Event Signal/1 -> setAttribute/1
  Clock/1 -> Timed to Event Signal/1
  connections:
  OUT_Commodity/RConn1 -- setAttribute/RConn1
  Source/RConn1 -- setAttribute/LConn1

== system Distribution_v2/Customer_12/Commodity_91 ==
  Clock : Clock
  Source : TimeBasedEntityGenerator  Distribution=Exponential  InitialSeed=18340  Mean=Mean  GenerateEntityAtSimulationStart=off
  Timed to Event Signal : TimedToEventSignal
  setAttribute : SetAttribute  AttributeName=Route|Origin|Destination|Start  AttributeFrom=Dialog|Dialog|Dialog|Signal port  AttributeValue="[12  22  13   0]|12|13|1"  AttributeTreatAsVector=0|1|1|1  EvaluatedAttributeValue="{[12  22  13   0];12;13;[]}"
      settings: InputPortMap=u3
  OUT_Commodity : PMIOPort  Port=1  Side=Right
  wires:
  Timed to Event Signal/1 -> setAttribute/1
  Clock/1 -> Timed to Event Signal/1
  connections:
  OUT_Commodity/RConn1 -- setAttribute/RConn1
  Source/RConn1 -- setAttribute/LConn1

== system Distribution_v2/Customer_13/Commodity_92 ==
  Clock : Clock
  Source : TimeBasedEntityGenerator  Distribution=Exponential  InitialSeed=18340  Mean=Mean  GenerateEntityAtSimulationStart=off
  Timed to Event Signal : TimedToEventSignal
  setAttribute : SetAttribute  AttributeName=Route|Origin|Destination|Start  AttributeFrom=Dialog|Dialog|Dialog|Signal port  AttributeValue="[13  22   1   0]|13|1|1"  AttributeTreatAsVector=0|1|1|1  EvaluatedAttributeValue="{[13  22   1   0];13;1;[]}"
      settings: InputPortMap=u3
  OUT_Commodity : PMIOPort  Port=1  Side=Right
  wires:
  Timed to Event Signal/1 -> setAttribute/1
  Clock/1 -> Timed to Event Signal/1
  connections:
  OUT_Commodity/RConn1 -- setAttribute/RConn1
  Source/RConn1 -- setAttribute/LConn1

== system Distribution_v2/Customer_13/Commodity_93 ==
  Clock : Clock
  Source : TimeBasedEntityGenerator  Distribution=Exponential  InitialSeed=18340  Mean=Mean  GenerateEntityAtSimulationStart=off
  Timed to Event Signal : TimedToEventSignal
  setAttribute : SetAttribute  AttributeName=Route|Origin|Destination|Start  AttributeFrom=Dialog|Dialog|Dialog|Signal port  AttributeValue="[13  22  18   6]|13|6|1"  AttributeTreatAsVector=0|1|1|1  EvaluatedAttributeValue="{[13  22  18   6];13;6;[]}"
      settings: InputPortMap=u3
  OUT_Commodity : PMIOPort  Port=1  Side=Right
  wires:
  Timed to Event Signal/1 -> setAttribute/1
  Clock/1 -> Timed to Event Signal/1
  connections:
  OUT_Commodity/RConn1 -- setAttribute/RConn1
  Source/RConn1 -- setAttribute/LConn1

== system Distribution_v2/Customer_13/Commodity_94 ==
  Clock : Clock
  Source : TimeBasedEntityGenerator  Distribution=Exponential  InitialSeed=18340  Mean=Mean  GenerateEntityAtSimulationStart=off
  Timed to Event Signal : TimedToEventSignal
  setAttribute : SetAttribute  AttributeName=Route|Origin|Destination|Start  AttributeFrom=Dialog|Dialog|Dialog|Signal port  AttributeValue="[13  22  20   8]|13|8|1"  AttributeTreatAsVector=0|1|1|1  EvaluatedAttributeValue="{[13  22  20   8];13;8;[]}"
      settings: InputPortMap=u3
  OUT_Commodity : PMIOPort  Port=1  Side=Right
  wires:
  Timed to Event Signal/1 -> setAttribute/1
  Clock/1 -> Timed to Event Signal/1
  connections:
  OUT_Commodity/RConn1 -- setAttribute/RConn1
  Source/RConn1 -- setAttribute/LConn1

== system Distribution_v2/Customer_13/Commodity_95 ==
  Clock : Clock
  Source : TimeBasedEntityGenerator  Distribution=Exponential  InitialSeed=18340  Mean=Mean  GenerateEntityAtSimulationStart=off
  Timed to Event Signal : TimedToEventSignal
  setAttribute : SetAttribute  AttributeName=Route|Origin|Destination|Start  AttributeFrom=Dialog|Dialog|Dialog|Signal port  AttributeValue="[13  22  18   9]|13|9|1"  AttributeTreatAsVector=0|1|1|1  EvaluatedAttributeValue="{[13  22  18   9];13;9;[]}"
      settings: InputPortMap=u3
  OUT_Commodity : PMIOPort  Port=1  Side=Right
  wires:
  Timed to Event Signal/1 -> setAttribute/1
  Clock/1 -> Timed to Event Signal/1
  connections:
  OUT_Commodity/RConn1 -- setAttribute/RConn1
  Source/RConn1 -- setAttribute/LConn1

== system Distribution_v2/Customer_13/Commodity_96 ==
  Clock : Clock
  Source : TimeBasedEntityGenerator  Distribution=Exponential  InitialSeed=18340  Mean=Mean  GenerateEntityAtSimulationStart=off
  Timed to Event Signal : TimedToEventSignal
  setAttribute : SetAttribute  AttributeName=Route|Origin|Destination|Start  AttributeFrom=Dialog|Dialog|Dialog|Signal port  AttributeValue="[13  22  12   0]|13|12|1"  AttributeTreatAsVector=0|1|1|1  EvaluatedAttributeValue="{[13  22  12   0];13;12;[]}"
      settings: InputPortMap=u3
  OUT_Commodity : PMIOPort  Port=1  Side=Right
  wires:
  Timed to Event Signal/1 -> setAttribute/1
  Clock/1 -> Timed to Event Signal/1
  connections:
  OUT_Commodity/RConn1 -- setAttribute/RConn1
  Source/RConn1 -- setAttribute/LConn1

== system Distribution_v2/Customer_13/Commodity_97 ==
  Clock : Clock
  Source : TimeBasedEntityGenerator  Distribution=Exponential  InitialSeed=18340  Mean=Mean  GenerateEntityAtSimulationStart=off
  Timed to Event Signal : TimedToEventSignal
  setAttribute : SetAttribute  AttributeName=Route|Origin|Destination|Start  AttributeFrom=Dialog|Dialog|Dialog|Signal port  AttributeValue="[13  22  20  15]|13|15|1"  AttributeTreatAsVector=0|1|1|1  EvaluatedAttributeValue="{[13  22  20  15];13;15;[]}"
      settings: InputPortMap=u3
  OUT_Commodity : PMIOPort  Port=1  Side=Right
  wires:
  Timed to Event Signal/1 -> setAttribute/1
  Clock/1 -> Timed to Event Signal/1
  connections:
  OUT_Commodity/RConn1 -- setAttribute/RConn1
  Source/RConn1 -- setAttribute/LConn1

== system Distribution_v2/Customer_14/Commodity_100 ==
  Clock : Clock
  Source : TimeBasedEntityGenerator  Distribution=Exponential  InitialSeed=18340  Mean=Mean  GenerateEntityAtSimulationStart=off
  Timed to Event Signal : TimedToEventSignal
  setAttribute : SetAttribute  AttributeName=Route|Origin|Destination|Start  AttributeFrom=Dialog|Dialog|Dialog|Signal port  AttributeValue="[14  20  18   4]|14|4|1"  AttributeTreatAsVector=0|1|1|1  EvaluatedAttributeValue="{[14  20  18   4];14;4;[]}"
      settings: InputPortMap=u3
  OUT_Commodity : PMIOPort  Port=1  Side=Right
  wires:
  Timed to Event Signal/1 -> setAttribute/1
  Clock/1 -> Timed to Event Signal/1
  connections:
  OUT_Commodity/RConn1 -- setAttribute/RConn1
  Source/RConn1 -- setAttribute/LConn1

== system Distribution_v2/Customer_14/Commodity_101 ==
  Clock : Clock
  Source : TimeBasedEntityGenerator  Distribution=Exponential  InitialSeed=18340  Mean=Mean  GenerateEntityAtSimulationStart=off
  Timed to Event Signal : TimedToEventSignal
  setAttribute : SetAttribute  AttributeName=Route|Origin|Destination|Start  AttributeFrom=Dialog|Dialog|Dialog|Signal port  AttributeValue="[14  20  22   5]|14|5|1"  AttributeTreatAsVector=0|1|1|1  EvaluatedAttributeValue="{[14  20  22   5];14;5;[]}"
      settings: InputPortMap=u3
  OUT_Commodity : PMIOPort  Port=1  Side=Right
  wires:
  Timed to Event Signal/1 -> setAttribute/1
  Clock/1 -> Timed to Event Signal/1
  connections:
  OUT_Commodity/RConn1 -- setAttribute/RConn1
  Source/RConn1 -- setAttribute/LConn1

== system Distribution_v2/Customer_14/Commodity_102 ==
  Clock : Clock
  Source : TimeBasedEntityGenerator  Distribution=Exponential  InitialSeed=18340  Mean=Mean  GenerateEntityAtSimulationStart=off
  Timed to Event Signal : TimedToEventSignal
  setAttribute : SetAttribute  AttributeName=Route|Origin|Destination|Start  AttributeFrom=Dialog|Dialog|Dialog|Signal port  AttributeValue="[14  20  18   6]|14|6|1"  AttributeTreatAsVector=0|1|1|1  EvaluatedAttributeValue="{[14  20  18   6];14;6;[]}"
      settings: InputPortMap=u3
  OUT_Commodity : PMIOPort  Port=1  Side=Right
  wires:
  Timed to Event Signal/1 -> setAttribute/1
  Clock/1 -> Timed to Event Signal/1
  connections:
  OUT_Commodity/RConn1 -- setAttribute/RConn1
  Source/RConn1 -- setAttribute/LConn1

== system Distribution_v2/Customer_14/Commodity_103 ==
  Clock : Clock
  Source : TimeBasedEntityGenerator  Distribution=Exponential  InitialSeed=18340  Mean=Mean  GenerateEntityAtSimulationStart=off
  Timed to Event Signal : TimedToEventSignal
  setAttribute : SetAttribute  AttributeName=Route|Origin|Destination|Start  AttributeFrom=Dialog|Dialog|Dialog|Signal port  AttributeValue="[14  20  18   9]|14|9|1"  AttributeTreatAsVector=0|1|1|1  EvaluatedAttributeValue="{[14  20  18   9];14;9;[]}"
      settings: InputPortMap=u3
  OUT_Commodity : PMIOPort  Port=1  Side=Right
  wires:
  Timed to Event Signal/1 -> setAttribute/1
  Clock/1 -> Timed to Event Signal/1
  connections:
  OUT_Commodity/RConn1 -- setAttribute/RConn1
  Source/RConn1 -- setAttribute/LConn1

== system Distribution_v2/Customer_14/Commodity_104 ==
  Clock : Clock
  Source : TimeBasedEntityGenerator  Distribution=Exponential  InitialSeed=18340  Mean=Mean  GenerateEntityAtSimulationStart=off
  Timed to Event Signal : TimedToEventSignal
  setAttribute : SetAttribute  AttributeName=Route|Origin|Destination|Start  AttributeFrom=Dialog|Dialog|Dialog|Signal port  AttributeValue="[14  20  22  10]|14|10|1"  AttributeTreatAsVector=0|1|1|1  EvaluatedAttributeValue="{[14  20  22  10];14;10;[]}"
      settings: InputPortMap=u3
  OUT_Commodity : PMIOPort  Port=1  Side=Right
  wires:
  Timed to Event Signal/1 -> setAttribute/1
  Clock/1 -> Timed to Event Signal/1
  connections:
  OUT_Commodity/RConn1 -- setAttribute/RConn1
  Source/RConn1 -- setAttribute/LConn1

== system Distribution_v2/Customer_14/Commodity_105 ==
  Clock : Clock
  Source : TimeBasedEntityGenerator  Distribution=Exponential  InitialSeed=18340  Mean=Mean  GenerateEntityAtSimulationStart=off
  Timed to Event Signal : TimedToEventSignal
  setAttribute : SetAttribute  AttributeName=Route|Origin|Destination|Start  AttributeFrom=Dialog|Dialog|Dialog|Signal port  AttributeValue="[14  20  22  13]|14|13|1"  AttributeTreatAsVector=0|1|1|1  EvaluatedAttributeValue="{[14  20  22  13];14;13;[]}"
      settings: InputPortMap=u3
  OUT_Commodity : PMIOPort  Port=1  Side=Right
  wires:
  Timed to Event Signal/1 -> setAttribute/1
  Clock/1 -> Timed to Event Signal/1
  connections:
  OUT_Commodity/RConn1 -- setAttribute/RConn1
  Source/RConn1 -- setAttribute/LConn1

== system Distribution_v2/Customer_14/Commodity_106 ==
  Clock : Clock
  Source : TimeBasedEntityGenerator  Distribution=Exponential  InitialSeed=18340  Mean=Mean  GenerateEntityAtSimulationStart=off
  Timed to Event Signal : TimedToEventSignal
  setAttribute : SetAttribute  AttributeName=Route|Origin|Destination|Start  AttributeFrom=Dialog|Dialog|Dialog|Signal port  AttributeValue="[14  20  15   0]|14|15|1"  AttributeTreatAsVector=0|1|1|1  EvaluatedAttributeValue="{[14  20  15   0];14;15;[]}"
      settings: InputPortMap=u3
  OUT_Commodity : PMIOPort  Port=1  Side=Right
  wires:
  Timed to Event Signal/1 -> setAttribute/1
  Clock/1 -> Timed to Event Signal/1
  connections:
  OUT_Commodity/RConn1 -- setAttribute/RConn1
  Source/RConn1 -- setAttribute/LConn1

== system Distribution_v2/Customer_14/Commodity_98 ==
  Clock : Clock
  Source : TimeBasedEntityGenerator  Distribution=Exponential  InitialSeed=18340  Mean=Mean  GenerateEntityAtSimulationStart=off
  Timed to Event Signal : TimedToEventSignal
  setAttribute : SetAttribute  AttributeName=Route|Origin|Destination|Start  AttributeFrom=Dialog|Dialog|Dialog|Signal port  AttributeValue="[14  20  18   2]|14|2|1"  AttributeTreatAsVector=0|1|1|1  EvaluatedAttributeValue="{[14  20  18   2];14;2;[]}"
      settings: InputPortMap=u3
  OUT_Commodity : PMIOPort  Port=1  Side=Right
  wires:
  Timed to Event Signal/1 -> setAttribute/1
  Clock/1 -> Timed to Event Signal/1
  connections:
  OUT_Commodity/RConn1 -- setAttribute/RConn1
  Source/RConn1 -- setAttribute/LConn1

== system Distribution_v2/Customer_14/Commodity_99 ==
  Clock : Clock
  Source : TimeBasedEntityGenerator  Distribution=Exponential  InitialSeed=18340  Mean=Mean  GenerateEntityAtSimulationStart=off
  Timed to Event Signal : TimedToEventSignal
  setAttribute : SetAttribute  AttributeName=Route|Origin|Destination|Start  AttributeFrom=Dialog|Dialog|Dialog|Signal port  AttributeValue="[14  20   3   0]|14|3|1"  AttributeTreatAsVector=0|1|1|1  EvaluatedAttributeValue="{[14  20   3   0];14;3;[]}"
      settings: InputPortMap=u3
  OUT_Commodity : PMIOPort  Port=1  Side=Right
  wires:
  Timed to Event Signal/1 -> setAttribute/1
  Clock/1 -> Timed to Event Signal/1
  connections:
  OUT_Commodity/RConn1 -- setAttribute/RConn1
  Source/RConn1 -- setAttribute/LConn1

== system Distribution_v2/Customer_15/Commodity_107 ==
  Clock : Clock
  Source : TimeBasedEntityGenerator  Distribution=Exponential  InitialSeed=18340  Mean=Mean  GenerateEntityAtSimulationStart=off
  Timed to Event Signal : TimedToEventSignal
  setAttribute : SetAttribute  AttributeName=Route|Origin|Destination|Start  AttributeFrom=Dialog|Dialog|Dialog|Signal port  AttributeValue="[15  20  22   5]|15|5|1"  AttributeTreatAsVector=0|1|1|1  EvaluatedAttributeValue="{[15  20  22   5];15;5;[]}"
      settings: InputPortMap=u3
  OUT_Commodity : PMIOPort  Port=1  Side=Right
  wires:
  Timed to Event Signal/1 -> setAttribute/1
  Clock/1 -> Timed to Event Signal/1
  connections:
  OUT_Commodity/RConn1 -- setAttribute/RConn1
  Source/RConn1 -- setAttribute/LConn1

== system Distribution_v2/Customer_15/Commodity_108 ==
  Clock : Clock
  Source : TimeBasedEntityGenerator  Distribution=Exponential  InitialSeed=18340  Mean=Mean  GenerateEntityAtSimulationStart=off
  Timed to Event Signal : TimedToEventSignal
  setAttribute : SetAttribute  AttributeName=Route|Origin|Destination|Start  AttributeFrom=Dialog|Dialog|Dialog|Signal port  AttributeValue="[15  20   7   0]|15|7|1"  AttributeTreatAsVector=0|1|1|1  EvaluatedAttributeValue="{[15  20   7   0];15;7;[]}"
      settings: InputPortMap=u3
  OUT_Commodity : PMIOPort  Port=1  Side=Right
  wires:
  Timed to Event Signal/1 -> setAttribute/1
  Clock/1 -> Timed to Event Signal/1
  connections:
  OUT_Commodity/RConn1 -- setAttribute/RConn1
  Source/RConn1 -- setAttribute/LConn1
